simulink model "xplane_tests"  (R2025b)
settings: Solver=ode4  StartTime=0.0  StopTime=600  FixedStep=0.05  RelTol=1e-3
StartFcn:
  | ins_initial_state_xplane_test;
StopFcn:
  | close_xplane;
values from neighbouring files (symbols this model uses):
  h_ref = 500    [tests_inicializar_xplane.m]
  VT_ref = 30    [tests_inicializar_xplane.m]
undefined symbols (not defined in the file or in its folder): C_alt, C_phi, C_theta, C_vel, Kp_sas, Kq, Kr, TrimInput, Xe
libraries: slpidlib x4
settings Model: Creator=Kaue  LastModifiedBy=julio

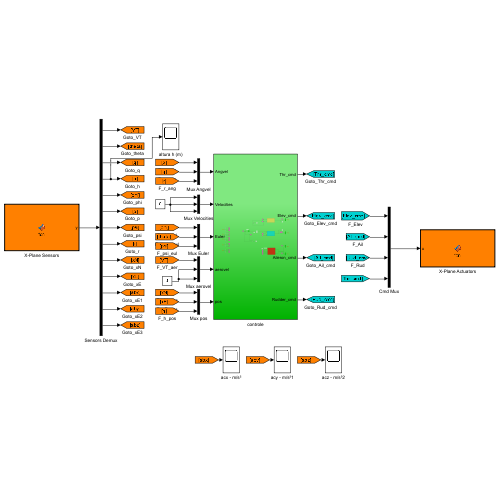
[thumbnail: Simulink's stored preview of the top-level diagram]
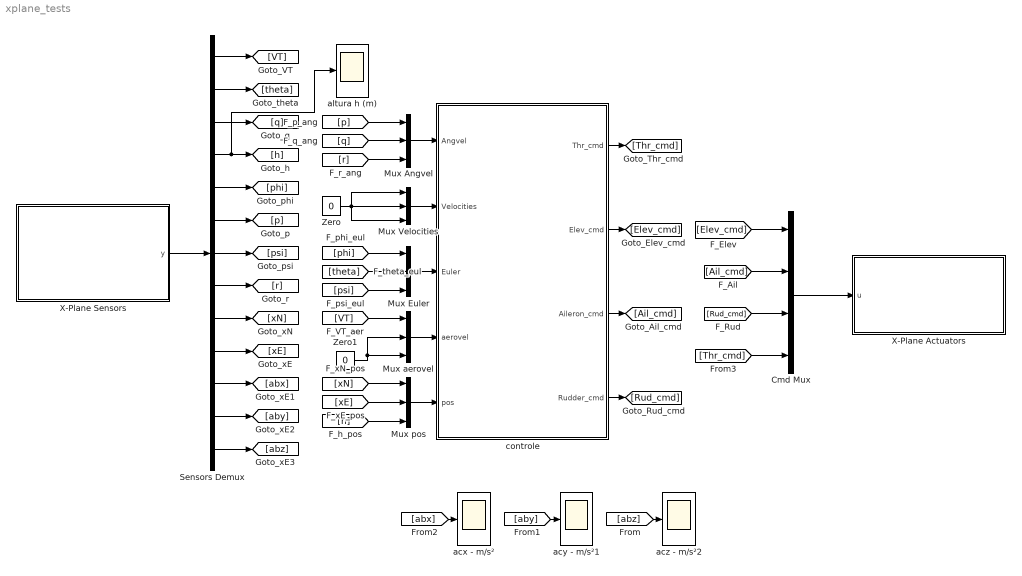
== system xplane_tests ==
  Cmd Mux : Mux
  Mux Angvel : Mux  Inputs=3
  Mux Euler : Mux  Inputs=3
  Mux Velocities : Mux  Inputs=3
  Mux aerovel : Mux  Inputs=3
  Mux pos : Mux  Inputs=3
  Sensors Demux : Demux  Outputs=13
  X-Plane Actuators : MATLAB Function  TreatAsAtomicUnit=on
  X-Plane Sensors : MATLAB Function  TreatAsAtomicUnit=on
  Zero : Constant  Value=0
  Zero1 : Constant  Value=0
  acx - m/s² : Scope
      settings: ActiveDisplayYMinimum=-2.4493518417362932  ActiveDisplayYMaximum=3.5786223936156132
  acy - m/s²1 : Scope
      settings: ActiveDisplayYMinimum=-3.7015716848387918  ActiveDisplayYMaximum=5.1695977106358137  DataLoggingVariableName=ScopeData8
  acz - m/s²2 : Scope
      settings: ActiveDisplayYMinimum=-7.1961969101845957  ActiveDisplayYMaximum=8.332036646245907  DataLoggingVariableName=ScopeData9
  altura h (m) : Scope
      settings: ActiveDisplayYMinimum=493.79105758666992  ActiveDisplayYMaximum=503.1589241027832  DataLoggingVariableName=ScopeData7
  controle : Subsystem
  wires:
  X-Plane Sensors/1(y) -> Sensors Demux/1
  Sensors Demux/1 -> [VT]
  Sensors Demux/2 -> [theta]
  Sensors Demux/3 -> [q]
  Sensors Demux/4 -> altura h (m)/1, [h]
  Sensors Demux/5 -> [phi]
  Sensors Demux/6 -> [p]
  Sensors Demux/7 -> [psi]
  Sensors Demux/8 -> [r]
  Sensors Demux/9 -> [xN]
  Sensors Demux/10 -> [xE]
  [p] -> Mux Angvel/1
  [q] -> Mux Angvel/2
  [r] -> Mux Angvel/3
  Mux Angvel/1 -> controle/1(Angvel)
  Zero/1 -> Mux Velocities/1, Mux Velocities/3, Mux Velocities/2
  Mux Velocities/1 -> controle/2(Velocities)
  [phi] -> Mux Euler/1
  [theta] -> Mux Euler/2
  [psi] -> Mux Euler/3
  Mux Euler/1 -> controle/3(Euler)
  [VT] -> Mux aerovel/1
  Mux aerovel/1 -> controle/4(aerovel)
  [xN] -> Mux pos/1
  [xE] -> Mux pos/2
  [h] -> Mux pos/3
  Mux pos/1 -> controle/5(pos)
  controle/1(Thr_cmd) -> [Thr_cmd]
  controle/2(Elev_cmd) -> [Elev_cmd]
  controle/3(Aileron_cmd) -> [Ail_cmd]
  controle/4(Rudder_cmd) -> [Rud_cmd]
  [Elev_cmd] -> Cmd Mux/1
  [Ail_cmd] -> Cmd Mux/2
  [Rud_cmd] -> Cmd Mux/3
  Cmd Mux/1 -> X-Plane Actuators/1(u)
  Zero1/1 -> Mux aerovel/2, Mux aerovel/3
  Sensors Demux/11 -> [abx]
  Sensors Demux/12 -> [aby]
  Sensors Demux/13 -> [abz]
  [abx] -> acx - m/s²/1
  [aby] -> acy - m/s²1/1
  [abz] -> acz - m/s²2/1
  [Thr_cmd] -> Cmd Mux/4

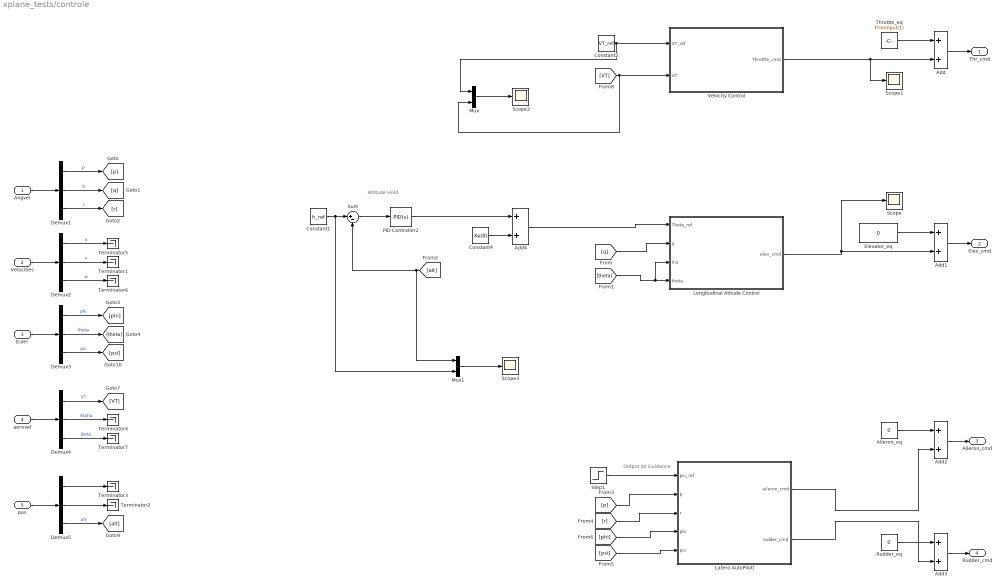
== system xplane_tests/controle ==
  note: Output do Guidance
  note: Altitude Hold
  Angvel : Inport
  Velocities : Inport  Port=2
  Euler : Inport  Port=3
  aerovel : Inport  Port=4
  pos : Inport  Port=5
  Add{,1..4} (5 alike) : Sum
  Aileron_eq : Constant  Value=0
  Constant1 : Constant  Value=h_ref
  Constant2 : Constant  Value=VT_ref
  Constant4 : Constant  Value=Xe(8)
  Demux{1..5} (5 alike) : Demux  Outputs=3
  Elevator_eq : Constant  Value=0
  Latero AutoPilotl : Subsystem
  Longitudinal Atitude Control : Subsystem
  Mux : Mux  Inputs=2
  Mux1 : Mux  Inputs=2
  PID Controller2 : slpidlib/PID Controller  Controller=PID  Form=Parallel  TimeDomain=Continuous-time  UseExternalTs=off  SampleTime=-1  IntegratorMethod=Forward Euler  FilterMethod=Forward Euler  ControllerParametersSource=internal  P=C_alt.Kp  I=C_alt.Ki  UseKiTs=off  D=C_alt.Kd  UseExternalDerivativeSource=off  N=C_alt.N  UseFilter=on  TunerSelectOption=Transfer Function Based (PID Tuner App)  InitialConditionSource=internal  InitialConditionForIntegrator=0  InitialConditionForFilter=0  DifferentiatorICPrevScaledInput=0  ExternalReset=none  TrackingMode=off  Kt=1  LimitOutput=on  SatLimitsSource=internal  UpperSaturationLimit=0.26  LowerSaturationLimit=-0.17  LinearizeAsGain=on  AntiWindupMode=clamping  Kb=1  LimitIntegrator=off  UpperIntegratorSaturationLimit=inf  LowerIntegratorSaturationLimit=-inf  POutMin=[]  POutMax=[]  IOutMin=[]  IOutMax=[]  DOutMin=[]  DOutMax=[]  NOutMin=[]  NOutMax=[]  SumOutMin=[]  SumOutMax=[]  SaturationOutMin=[]  SaturationOutMax=[]  PParamMin=[]  PParamMax=[]  IParamMin=[]  IParamMax=[]  DParamMin=[]  DParamMax=[]  NParamMin=[]  NParamMax=[]  KbParamMin=[]  KbParamMax=[]  KtParamMin=[]  KtParamMax=[]  KbOutMin=[]  KbOutMax=[]  KtOutMin=[]  KtOutMax=[]  IntegratorOutMin=[]  IntegratorOutMax=[]  FilterOutMin=[]  FilterOutMax=[]  SumI1OutMin=[]  SumI1OutMax=[]  SumI2OutMin=[]  SumI2OutMax=[]  SumI3OutMin=[]  SumI3OutMax=[]  SumI4OutMin=[]  SumI4OutMax=[]  SumDOutMin=[]  SumDOutMax=[]  DifferentiatorOutMin=[]  DifferentiatorOutMax=[]  FilterDiffOutCoefMin=[]  FilterDiffOutCoefMax=[]  ReciprocalOutMin=[]  ReciprocalOutMax=[]  SumDenOutMin=[]  SumDenOutMax=[]  SumNumOutMin=[]  SumNumOutMax=[]  DivideOutMin=[]  DivideOutMax=[]  UdiffTsProdOutMin=[]  UdiffTsProdOutMax=[]  NTsProdOutMin=[]  NTsProdOutMax=[]  UintegralTsProdOutMin=[]  UintegralTsProdOutMax=[]  UngainTsProdOutMin=[]  UngainTsProdOutMax=[]  ClampingZeroOutDataTypeStr=Inherit: Inherit via back propagation  ClampingZeroOutMin=[]  ClampingZeroOutMax=[]  FilterDenConstantOutDataTypeStr=Inherit: Inherit via back propagation  FilterDenConstantOutMin=[]  FilterDenConstantOutMax=[]  PCopyOutDataTypeStr=Inherit: Inherit via back propagation  PCopyOutMin=[]  PCopyOutMax=[]  NCopyOutDataTypeStr=Inherit: Inherit via back propagation  NCopyOutMin=[]  NCopyOutMax=[]  IntegratorContinuousStateAttributes=''  IntegratorStateMustResolveToSignalObject=off  IntegratorRTWStateStorageClass=Auto  FilterContinuousStateAttributes=''  FilterStateMustResolveToSignalObject=off  FilterRTWStateStorageClass=Auto  ParallelPVariant=InternalParameters  IdealPVariant=Disabled  IVariant=InternalParameters  DVariant=InternalParameters  IntegratorVariant=Continuous  SatVariant=Enabled  AWVariant=ContClampingParallel  PCopyVariant=Disabled  TRVariant=Disabled  FdbkBlocksVariant=Forward  IdealPFdbkVariant=Disabled  SatFdbkVariant=Disabled  DerivativeFilterVariant=ContFilter  NVariant=InternalParameters  NCopyVariant=Disabled  FilterICVariant=InternalICsFilter  IntegratorICVariant=InternalICs  ExternalResetVariant=Disabled  TRSumVariant=Passthrough  SumFdbkVariant=Disabled  SumVariant=Sum_PID  TsampFilterVariant=InternalTs  TsampNgainVariant=Passthrough  TsampIntegralVariant=Disabled_SignalSpec  ExternalSaturationOutDataTypeStr=Inherit: Same as second input  DerivativeSourceVariant=ErrorSignal  PreIntVariant=InternalPreInt
  Rudder_eq : Constant  Value=0
  Scope{,1..3} (4 alike) : Scope
      Scope settings: ActiveDisplayYMinimum=-1E-5  ActiveDisplayYMaximum=0.0001
      Scope1 settings: ActiveDisplayYMinimum=-746.9186  ActiveDisplayYMaximum=116.1605  DataLoggingVariableName=ScopeData2
      Scope2 settings: ActiveDisplayYMinimum=-70.825855594492936  ActiveDisplayYMaximum=79.160614638107518  DataLoggingVariableName=ScopeData4
      Scope3 settings: ActiveDisplayYMinimum=-113.29137312954269  ActiveDisplayYMaximum=148.47510576001991  DataLoggingVariableName=ScopeData6
  Step1 : Step  Time=5  After=deg2rad(20)  SampleTime=0
  Sum : Sum  Inputs=|+-
  Terminator{1..7} (7 alike) : Terminator
  Throttle_eq : Constant  Value=TrimInput(1)
  Velocity Control : Subsystem
  Thr_cmd : Outport
  Elev_cmd : Outport  Port=2
  Aileron_cmd : Outport  Port=3
  Rudder_cmd : Outport  Port=4
  wires:
  Constant2/1 -> Velocity Control/1(VT_ref), Mux/1
  PID Controller2/1 -> Add4/1
  Sum/1 -> PID Controller2/1
  Mux1/1 -> Scope3/1
  Throttle_eq/1 -> Add/1
  Add3/1 -> Rudder_cmd/1
  Add2/1 -> Aileron_cmd/1
  Latero AutoPilotl/2(rudder_cmd) -> Add3/2
  Aileron_eq/1 -> Add2/1
  Rudder_eq/1 -> Add3/1
  Elevator_eq/1 -> Add1/1
  Latero AutoPilotl/1(aileron_cmd) -> Add2/2
  Velocity Control/1(Throttle_cmd) -> Add/2, Scope1/1
  Add/1 -> Thr_cmd/1
  Longitudinal Atitude Control/1(elev_cmd) -> Add1/2, Scope/1
  Add1/1 -> Elev_cmd/1
  Mux/1 -> Scope2/1
  Constant1/1 -> Sum/1, Mux1/2
  Step1/1 -> Latero AutoPilotl/1(psi_ref)
  Add4/1 -> Longitudinal Atitude Control/1(Theta_ref)
  Constant4/1 -> Add4/2
  [phi] -> Latero AutoPilotl/4(phi)
  [psi] -> Latero AutoPilotl/5(psi)
  [r] -> Latero AutoPilotl/3(r)
  [p] -> Latero AutoPilotl/2(p)
  [alt] -> Mux1/1, Sum/2
  Demux5/1 -> Terminator3/1
  Demux5/2 -> Terminator2/1
  Demux5/3 -> [alt]  "alt"
  pos/1 -> Demux5/1
  [VT] -> Velocity Control/2(VT), Mux/2
  [q] -> Longitudinal Atitude Control/2(q)
  Demux4/3 -> Terminator7/1  "Beta"
  Demux4/2 -> Terminator4/1  "Alpha"
  Demux4/1 -> [VT]  "VT"
  aerovel/1 -> Demux4/1
  [theta] -> Longitudinal Atitude Control/4(theta), Longitudinal Atitude Control/3(In3)
  Demux2/2 -> Terminator1/1  "v"
  Demux2/1 -> Terminator5/1  "u"
  Demux2/3 -> Terminator6/1  "w"
  Demux3/2 -> [theta]  "theta"
  Demux3/1 -> [phi]  "phi"
  Demux3/3 -> [psi]  "psi"
  Euler/1 -> Demux3/1
  Demux1/3 -> [r]  "r"
  Demux1/2 -> [q]  "q"
  Demux1/1 -> [p]  "p"
  Velocities/1 -> Demux2/1
  Angvel/1 -> Demux1/1

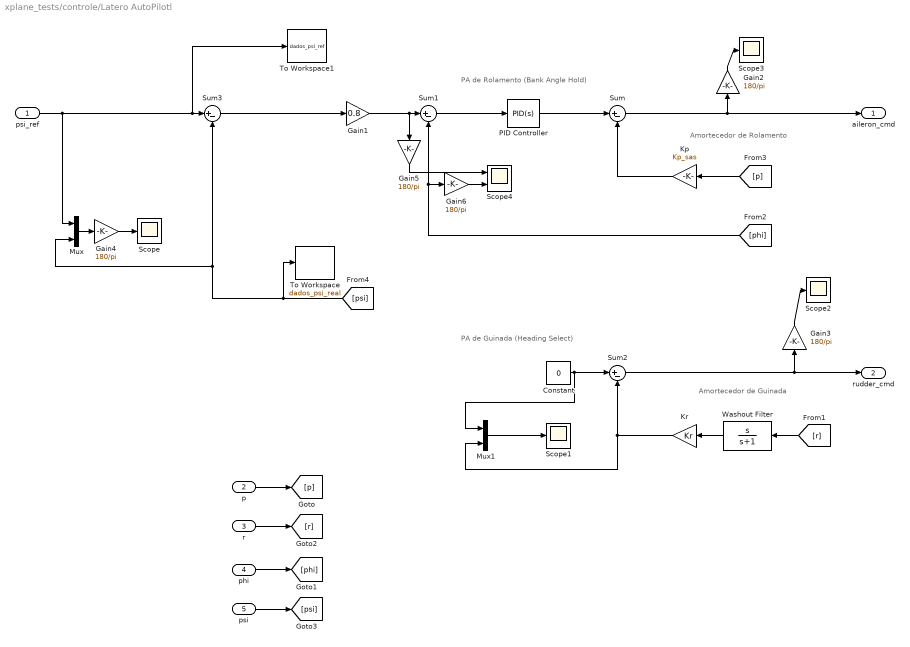
== system xplane_tests/controle/Latero AutoPilotl ==
  note: PA de Guinada (Heading Select)
  note: Amortecedor de Guinada
  note: Amortecedor de Rolamento
  note: PA de Rolamento (Bank Angle Hold)
  psi_ref : Inport
  p : Inport  Port=2
  r : Inport  Port=3
  phi : Inport  Port=4
  psi : Inport  Port=5
  Constant : Constant  Value=0
  Gain1 : Gain  Gain=0.8
  Gain{2..6} (5 alike) : Gain  Gain=180/pi
  Kp : Gain  Gain=Kp_sas
  Kr : Gain  Gain=Kr
  Mux : Mux  Inputs=2
  Mux1 : Mux  Inputs=2
  PID Controller : slpidlib/PID Controller  Controller=PID  Form=Parallel  TimeDomain=Continuous-time  UseExternalTs=off  SampleTime=-1  IntegratorMethod=Forward Euler  FilterMethod=Forward Euler  ControllerParametersSource=internal  P=C_phi.Kp  I=C_phi.Ki  UseKiTs=off  D=C_phi.Kd  UseExternalDerivativeSource=off  N=C_phi.N  UseFilter=on  TunerSelectOption=Transfer Function Based (PID Tuner App)  InitialConditionSource=internal  InitialConditionForIntegrator=0  InitialConditionForFilter=0  DifferentiatorICPrevScaledInput=0  ExternalReset=none  TrackingMode=off  Kt=1  LimitOutput=on  SatLimitsSource=internal  UpperSaturationLimit=0.4363  LowerSaturationLimit=-0.4363  LinearizeAsGain=on  AntiWindupMode=clamping  Kb=1  LimitIntegrator=off  UpperIntegratorSaturationLimit=inf  LowerIntegratorSaturationLimit=-inf  POutMin=[]  POutMax=[]  IOutMin=[]  IOutMax=[]  DOutMin=[]  DOutMax=[]  NOutMin=[]  NOutMax=[]  SumOutMin=[]  SumOutMax=[]  SaturationOutMin=[]  SaturationOutMax=[]  PParamMin=[]  PParamMax=[]  IParamMin=[]  IParamMax=[]  DParamMin=[]  DParamMax=[]  NParamMin=[]  NParamMax=[]  KbParamMin=[]  KbParamMax=[]  KtParamMin=[]  KtParamMax=[]  KbOutMin=[]  KbOutMax=[]  KtOutMin=[]  KtOutMax=[]  IntegratorOutMin=[]  IntegratorOutMax=[]  FilterOutMin=[]  FilterOutMax=[]  SumI1OutMin=[]  SumI1OutMax=[]  SumI2OutMin=[]  SumI2OutMax=[]  SumI3OutMin=[]  SumI3OutMax=[]  SumI4OutMin=[]  SumI4OutMax=[]  SumDOutMin=[]  SumDOutMax=[]  DifferentiatorOutMin=[]  DifferentiatorOutMax=[]  FilterDiffOutCoefMin=[]  FilterDiffOutCoefMax=[]  ReciprocalOutMin=[]  ReciprocalOutMax=[]  SumDenOutMin=[]  SumDenOutMax=[]  SumNumOutMin=[]  SumNumOutMax=[]  DivideOutMin=[]  DivideOutMax=[]  UdiffTsProdOutMin=[]  UdiffTsProdOutMax=[]  NTsProdOutMin=[]  NTsProdOutMax=[]  UintegralTsProdOutMin=[]  UintegralTsProdOutMax=[]  UngainTsProdOutMin=[]  UngainTsProdOutMax=[]  ClampingZeroOutDataTypeStr=Inherit: Inherit via back propagation  ClampingZeroOutMin=[]  ClampingZeroOutMax=[]  FilterDenConstantOutDataTypeStr=Inherit: Inherit via back propagation  FilterDenConstantOutMin=[]  FilterDenConstantOutMax=[]  PCopyOutDataTypeStr=Inherit: Inherit via back propagation  PCopyOutMin=[]  PCopyOutMax=[]  NCopyOutDataTypeStr=Inherit: Inherit via back propagation  NCopyOutMin=[]  NCopyOutMax=[]  IntegratorContinuousStateAttributes=''  IntegratorStateMustResolveToSignalObject=off  IntegratorRTWStateStorageClass=Auto  FilterContinuousStateAttributes=''  FilterStateMustResolveToSignalObject=off  FilterRTWStateStorageClass=Auto  ParallelPVariant=InternalParameters  IdealPVariant=Disabled  IVariant=InternalParameters  DVariant=InternalParameters  IntegratorVariant=Continuous  SatVariant=Enabled  AWVariant=ContClampingParallel  PCopyVariant=Disabled  TRVariant=Disabled  FdbkBlocksVariant=Forward  IdealPFdbkVariant=Disabled  SatFdbkVariant=Disabled  DerivativeFilterVariant=ContFilter  NVariant=InternalParameters  NCopyVariant=Disabled  FilterICVariant=InternalICsFilter  IntegratorICVariant=InternalICs  ExternalResetVariant=Disabled  TRSumVariant=Passthrough  SumFdbkVariant=Disabled  SumVariant=Sum_PID  TsampFilterVariant=InternalTs  TsampNgainVariant=Passthrough  TsampIntegralVariant=Disabled_SignalSpec  ExternalSaturationOutDataTypeStr=Inherit: Same as second input  DerivativeSourceVariant=ErrorSignal  PreIntVariant=InternalPreInt
  Scope{,1..3} (4 alike) : Scope
      Scope settings: ActiveDisplayYMinimum=-9.73683  ActiveDisplayYMaximum=51.08187  DataLoggingVariableName=ScopeData5
      Scope1 settings: ActiveDisplayYMinimum=-0.53028169211297194  ActiveDisplayYMaximum=0.24100187800441716
      Scope2 settings: ActiveDisplayYMinimum=-4.64142  ActiveDisplayYMaximum=2.08449
      Scope3 settings: ActiveDisplayYMinimum=-384.74036  ActiveDisplayYMaximum=1108.75141  DataLoggingVariableName=ScopeData2
  Scope4 : Scope  NumInputPorts=2
      settings: ActiveDisplayYMinimum=-4.8655  ActiveDisplayYMaximum=43.78946  DataLoggingVariableName=ScopeData3
  Sum{,1..3} (4 alike) : Sum  Inputs=|+-
  To Workspace : ToWorkspace  VariableName=dados_psi_real  SaveFormat=Timeseries  SampleTime=-1
      settings: Save2DSignal=2-D array (concatenate along first dimension)
  To Workspace1 : ToWorkspace  VariableName=dados_psi_ref  SaveFormat=Timeseries  SampleTime=-1
      settings: Save2DSignal=2-D array (concatenate along first dimension)
  Washout Filter : TransferFcn  Numerator=[1 0]  Denominator=[1 1]
  aileron_cmd : Outport
  rudder_cmd : Outport  Port=2
  wires:
  Gain6/1 -> Scope4/2
  Gain5/1 -> Scope4/1
  Gain4/1 -> Scope/1
  Gain3/1 -> Scope2/1
  Gain2/1 -> Scope3/1
  Mux1/1 -> Scope1/1
  Mux/1 -> Gain4/1
  Gain1/1 -> Sum1/1, Gain5/1
  Constant/1 -> Sum2/1, Mux1/1
  Sum2/1 -> rudder_cmd/1, Gain3/1
  psi_ref/1 -> Sum3/1, To Workspace1/1, Mux/1
  [psi] -> Mux/2, Sum3/2, To Workspace/1
  Sum3/1 -> Gain1/1
  psi/1 -> [psi]
  phi/1 -> [phi]
  Washout Filter/1 -> Kr/1
  r/1 -> [r]
  Kr/1 -> Sum2/2, Mux1/2
  [r] -> Washout Filter/1
  p/1 -> [p]
  PID Controller/1 -> Sum/1
  Kp/1 -> Sum/2
  [phi] -> Gain6/1, Sum1/2
  [p] -> Kp/1
  Sum/1 -> aileron_cmd/1, Gain2/1
  Sum1/1 -> PID Controller/1

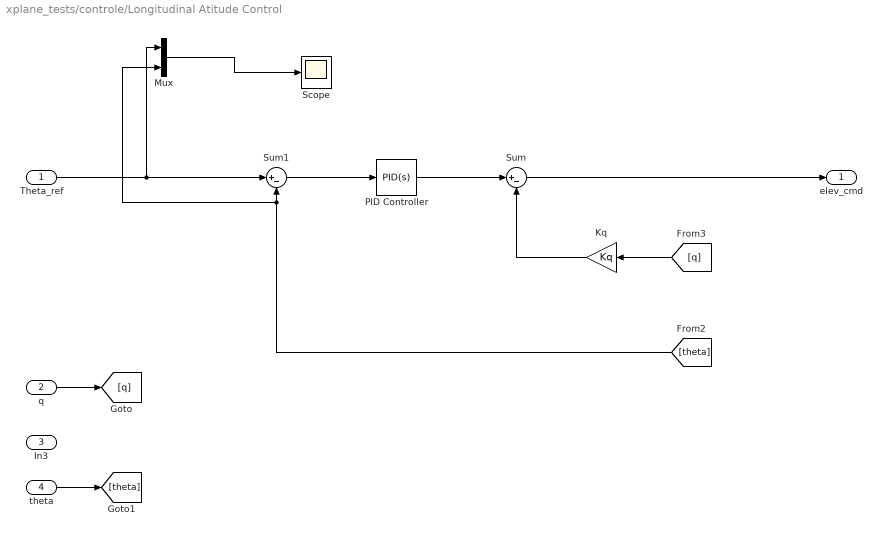
== system xplane_tests/controle/Longitudinal Atitude Control ==
  Theta_ref : Inport
  q : Inport  Port=2
  In3 : Inport  Port=3
  theta : Inport  Port=4
  Kq : Gain  Gain=Kq
  Mux : Mux  Inputs=2
  PID Controller : slpidlib/PID Controller  Controller=PID  Form=Parallel  TimeDomain=Continuous-time  UseExternalTs=off  SampleTime=-1  IntegratorMethod=Forward Euler  FilterMethod=Forward Euler  ControllerParametersSource=internal  P=C_theta.Kp  I=C_theta.Ki  UseKiTs=off  D=C_theta.Kd  UseExternalDerivativeSource=off  N=C_theta.N  UseFilter=on  TunerSelectOption=Transfer Function Based (PID Tuner App)  InitialConditionSource=internal  InitialConditionForIntegrator=0  InitialConditionForFilter=0  DifferentiatorICPrevScaledInput=0  ExternalReset=none  TrackingMode=off  Kt=1  LimitOutput=on  SatLimitsSource=internal  UpperSaturationLimit=0.4363  LowerSaturationLimit=-0.4363  LinearizeAsGain=on  AntiWindupMode=clamping  Kb=1  LimitIntegrator=off  UpperIntegratorSaturationLimit=inf  LowerIntegratorSaturationLimit=-inf  POutMin=[]  POutMax=[]  IOutMin=[]  IOutMax=[]  DOutMin=[]  DOutMax=[]  NOutMin=[]  NOutMax=[]  SumOutMin=[]  SumOutMax=[]  SaturationOutMin=[]  SaturationOutMax=[]  PParamMin=[]  PParamMax=[]  IParamMin=[]  IParamMax=[]  DParamMin=[]  DParamMax=[]  NParamMin=[]  NParamMax=[]  KbParamMin=[]  KbParamMax=[]  KtParamMin=[]  KtParamMax=[]  KbOutMin=[]  KbOutMax=[]  KtOutMin=[]  KtOutMax=[]  IntegratorOutMin=[]  IntegratorOutMax=[]  FilterOutMin=[]  FilterOutMax=[]  SumI1OutMin=[]  SumI1OutMax=[]  SumI2OutMin=[]  SumI2OutMax=[]  SumI3OutMin=[]  SumI3OutMax=[]  SumI4OutMin=[]  SumI4OutMax=[]  SumDOutMin=[]  SumDOutMax=[]  DifferentiatorOutMin=[]  DifferentiatorOutMax=[]  FilterDiffOutCoefMin=[]  FilterDiffOutCoefMax=[]  ReciprocalOutMin=[]  ReciprocalOutMax=[]  SumDenOutMin=[]  SumDenOutMax=[]  SumNumOutMin=[]  SumNumOutMax=[]  DivideOutMin=[]  DivideOutMax=[]  UdiffTsProdOutMin=[]  UdiffTsProdOutMax=[]  NTsProdOutMin=[]  NTsProdOutMax=[]  UintegralTsProdOutMin=[]  UintegralTsProdOutMax=[]  UngainTsProdOutMin=[]  UngainTsProdOutMax=[]  ClampingZeroOutDataTypeStr=Inherit: Inherit via back propagation  ClampingZeroOutMin=[]  ClampingZeroOutMax=[]  FilterDenConstantOutDataTypeStr=Inherit: Inherit via back propagation  FilterDenConstantOutMin=[]  FilterDenConstantOutMax=[]  PCopyOutDataTypeStr=Inherit: Inherit via back propagation  PCopyOutMin=[]  PCopyOutMax=[]  NCopyOutDataTypeStr=Inherit: Inherit via back propagation  NCopyOutMin=[]  NCopyOutMax=[]  IntegratorContinuousStateAttributes=''  IntegratorStateMustResolveToSignalObject=off  IntegratorRTWStateStorageClass=Auto  FilterContinuousStateAttributes=''  FilterStateMustResolveToSignalObject=off  FilterRTWStateStorageClass=Auto  ParallelPVariant=InternalParameters  IdealPVariant=Disabled  IVariant=InternalParameters  DVariant=InternalParameters  IntegratorVariant=Continuous  SatVariant=Enabled  AWVariant=ContClampingParallel  PCopyVariant=Disabled  TRVariant=Disabled  FdbkBlocksVariant=Forward  IdealPFdbkVariant=Disabled  SatFdbkVariant=Disabled  DerivativeFilterVariant=ContFilter  NVariant=InternalParameters  NCopyVariant=Disabled  FilterICVariant=InternalICsFilter  IntegratorICVariant=InternalICs  ExternalResetVariant=Disabled  TRSumVariant=Passthrough  SumFdbkVariant=Disabled  SumVariant=Sum_PID  TsampFilterVariant=InternalTs  TsampNgainVariant=Passthrough  TsampIntegralVariant=Disabled_SignalSpec  ExternalSaturationOutDataTypeStr=Inherit: Same as second input  DerivativeSourceVariant=ErrorSignal  PreIntVariant=InternalPreInt
  Scope : Scope
      settings: ActiveDisplayYMinimum=-0.22285  ActiveDisplayYMaximum=0.02179  DataLoggingVariableName=ScopeData3
  Sum : Sum  Inputs=|+-
  Sum1 : Sum  Inputs=|+-
  elev_cmd : Outport
  wires:
  Mux/1 -> Scope/1
  Theta_ref/1 -> Sum1/1, Mux/1
  q/1 -> [q]
  theta/1 -> [theta]
  PID Controller/1 -> Sum/1
  Kq/1 -> Sum/2
  [theta] -> Sum1/2, Mux/2
  [q] -> Kq/1
  Sum/1 -> elev_cmd/1
  Sum1/1 -> PID Controller/1

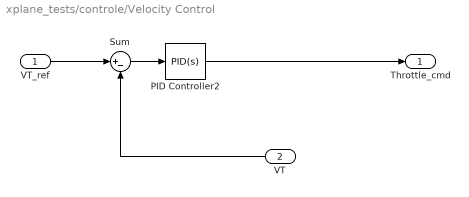
== system xplane_tests/controle/Velocity Control ==
  VT_ref : Inport
  VT : Inport  Port=2
  PID Controller2 : slpidlib/PID Controller  Controller=PID  Form=Parallel  TimeDomain=Continuous-time  UseExternalTs=off  SampleTime=-1  IntegratorMethod=Forward Euler  FilterMethod=Forward Euler  ControllerParametersSource=internal  P=C_vel.Kp  I=C_vel.Ki  UseKiTs=off  D=C_vel.Kd  UseExternalDerivativeSource=off  N=C_vel.N  UseFilter=on  TunerSelectOption=Transfer Function Based (PID Tuner App)  InitialConditionSource=internal  InitialConditionForIntegrator=0  InitialConditionForFilter=0  DifferentiatorICPrevScaledInput=0  ExternalReset=none  TrackingMode=off  Kt=1  LimitOutput=on  SatLimitsSource=internal  UpperSaturationLimit=0.51  LowerSaturationLimit=-0.49  LinearizeAsGain=on  AntiWindupMode=clamping  Kb=1  LimitIntegrator=off  UpperIntegratorSaturationLimit=inf  LowerIntegratorSaturationLimit=-inf  POutMin=[]  POutMax=[]  IOutMin=[]  IOutMax=[]  DOutMin=[]  DOutMax=[]  NOutMin=[]  NOutMax=[]  SumOutMin=[]  SumOutMax=[]  SaturationOutMin=[]  SaturationOutMax=[]  PParamMin=[]  PParamMax=[]  IParamMin=[]  IParamMax=[]  DParamMin=[]  DParamMax=[]  NParamMin=[]  NParamMax=[]  KbParamMin=[]  KbParamMax=[]  KtParamMin=[]  KtParamMax=[]  KbOutMin=[]  KbOutMax=[]  KtOutMin=[]  KtOutMax=[]  IntegratorOutMin=[]  IntegratorOutMax=[]  FilterOutMin=[]  FilterOutMax=[]  SumI1OutMin=[]  SumI1OutMax=[]  SumI2OutMin=[]  SumI2OutMax=[]  SumI3OutMin=[]  SumI3OutMax=[]  SumI4OutMin=[]  SumI4OutMax=[]  SumDOutMin=[]  SumDOutMax=[]  DifferentiatorOutMin=[]  DifferentiatorOutMax=[]  FilterDiffOutCoefMin=[]  FilterDiffOutCoefMax=[]  ReciprocalOutMin=[]  ReciprocalOutMax=[]  SumDenOutMin=[]  SumDenOutMax=[]  SumNumOutMin=[]  SumNumOutMax=[]  DivideOutMin=[]  DivideOutMax=[]  UdiffTsProdOutMin=[]  UdiffTsProdOutMax=[]  NTsProdOutMin=[]  NTsProdOutMax=[]  UintegralTsProdOutMin=[]  UintegralTsProdOutMax=[]  UngainTsProdOutMin=[]  UngainTsProdOutMax=[]  ClampingZeroOutDataTypeStr=Inherit: Inherit via back propagation  ClampingZeroOutMin=[]  ClampingZeroOutMax=[]  FilterDenConstantOutDataTypeStr=Inherit: Inherit via back propagation  FilterDenConstantOutMin=[]  FilterDenConstantOutMax=[]  PCopyOutDataTypeStr=Inherit: Inherit via back propagation  PCopyOutMin=[]  PCopyOutMax=[]  NCopyOutDataTypeStr=Inherit: Inherit via back propagation  NCopyOutMin=[]  NCopyOutMax=[]  IntegratorContinuousStateAttributes=''  IntegratorStateMustResolveToSignalObject=off  IntegratorRTWStateStorageClass=Auto  FilterContinuousStateAttributes=''  FilterStateMustResolveToSignalObject=off  FilterRTWStateStorageClass=Auto  ParallelPVariant=InternalParameters  IdealPVariant=Disabled  IVariant=InternalParameters  DVariant=InternalParameters  IntegratorVariant=Continuous  SatVariant=Enabled  AWVariant=ContClampingParallel  PCopyVariant=Disabled  TRVariant=Disabled  FdbkBlocksVariant=Forward  IdealPFdbkVariant=Disabled  SatFdbkVariant=Disabled  DerivativeFilterVariant=ContFilter  NVariant=InternalParameters  NCopyVariant=Disabled  FilterICVariant=InternalICsFilter  IntegratorICVariant=InternalICs  ExternalResetVariant=Disabled  TRSumVariant=Passthrough  SumFdbkVariant=Disabled  SumVariant=Sum_PID  TsampFilterVariant=InternalTs  TsampNgainVariant=Passthrough  TsampIntegralVariant=Disabled_SignalSpec  ExternalSaturationOutDataTypeStr=Inherit: Same as second input  DerivativeSourceVariant=ErrorSignal  PreIntVariant=InternalPreInt
  Sum : Sum  Inputs=|+-
  Throttle_cmd : Outport
  wires:
  Sum/1 -> PID Controller2/1
  VT_ref/1 -> Sum/1
  PID Controller2/1 -> Throttle_cmd/1
  VT/1 -> Sum/2

== matlab function xplane_tests/X-Plane Sensors ==
  settings: updateMethod=DISCRETE  sampleTime=0.05
  data: y output
function y = fcn()
%#codegen
coder.extrinsic('ins_read_xplane');
y = zeros(13,1);
tmp = zeros(1,13);
tmp = double(ins_read_xplane(0));
y(:) = tmp(:);
end

== matlab function xplane_tests/X-Plane Actuators ==
  settings: updateMethod=DISCRETE  sampleTime=0.05
  data: u input
function fcn(u)
%#codegen
coder.extrinsic('ins_send_xplane');
ins_send_xplane(u);
end
